simulink model "stateObserverControl"  (R2023b)
settings: Solver=VariableStepAuto  StartTime=0.0  StopTime=10  RelTol=1e-3
values from neighbouring files (symbols this model uses):
  K = Kaug(1:length(A))    [Controller.m]
  Km = Kaug(length(A)+1:end)    [Controller.m]
  L = place(A',C',poles)'    [Controller.m]
  Ma = [0 , 1 ; -1, 2*cos(w0)]    [Controller.m]
  Mb = [0;1]    [Controller.m]
  sys_est_ss = ss(A,B,C,D,Ts)    [Controller.m]
  Ts = 1/fs    (= 5e-05)    [Controller.m]
libraries: simulink x1
settings Model: Creator=NCS  LastModifiedBy=NCS

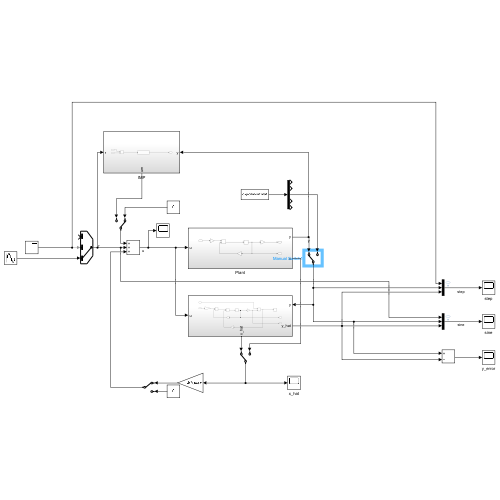
[thumbnail: Simulink's stored preview of the top-level diagram]
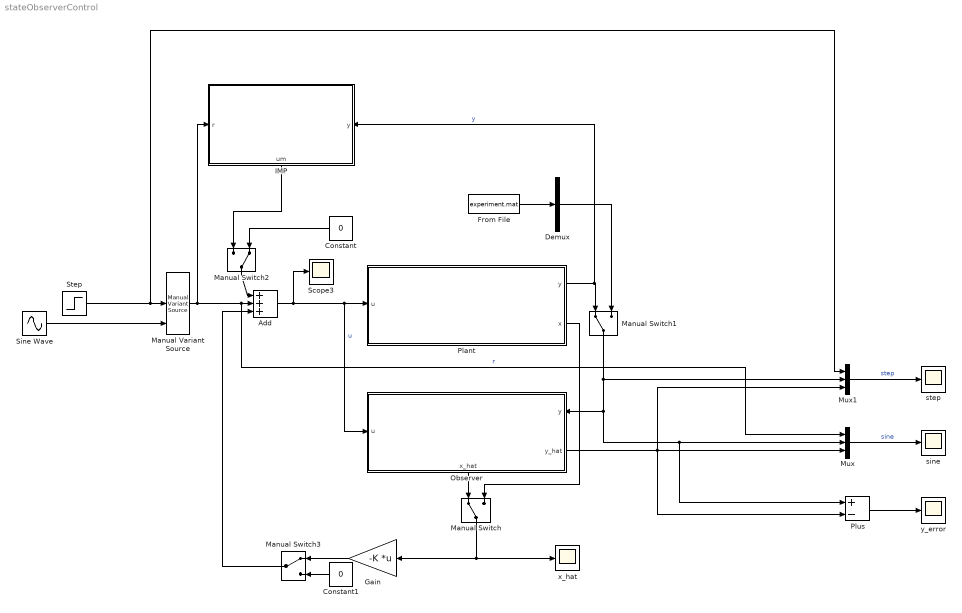
== system stateObserverControl ==
  Add : Sum  Inputs=+++
  Constant : Constant  Value=0
  Constant1 : Constant  Value=0
  Demux : Demux  Outputs=5
  From File : FromFile  FileName=experiment.mat  SampleTime=0
  Gain : Gain  Gain=-K  Multiplication=Matrix(K*u) (u vector)
  IMP : Subsystem
      settings: PortSchema="{\"entries\":[{\"content\":{\"sides\":[{\"content\":{\"connectorIds\":[\"In1\"]},\"type\":\"ConnectorPlacement.EquallySpacedRectSide\",\"uuid\":\"5d5e4b93-0997-4cc6-bb38-a0bc2c16a1b8\"},{\"content\":{\"connectorIds\":[\"In2\"],\"side\":\"RIGHT\"},\"type\":\"ConnectorPlacement.EquallySpacedRectSide\",\"uuid\":\"6a4a0bd4-0b0e-4fe8-aac6-62d10dbc348f\"},{\"content\":{\"side\":\"TOP\"},\"type\":\"ConnectorPlacement.EquallySpacedRectSide\",\"uuid\":\"dff729df-3d3e-4d9e-a17d-f1c4cc3cc1b7\"},{\"content\":{\"connectorIds\":[\"Out1\"],\"side\":\"BOTTOM\"},\"type\":\"ConnectorPlacement.EquallySpacedRectSide\",\"uuid\":\"a2ceeb7c-1f2e-4c64-a024-e96d715f5345\"}]},\"type\":\"ConnectorPlacement.EquallySpacedConnector\",\"uuid\":\"173e3c82-e772-4c04-9f4e-952750faad31\"}],\"packageUris\":[\"http://schema.mathworks.com/mf0/Connector/R2020b\"],\"version\":\"1.0\"}"
  Manual Variant Source : simulink/Signal Routing/Manual Variant Source  NumChoices=3  LabelModeActiveChoice=V_3
  Manual Switch : ManualSwitch
  Manual Switch1 : ManualSwitch
  Manual Switch2 : ManualSwitch  CurrentSetting=0
  Manual Switch3 : ManualSwitch
  Mux : Mux  Inputs=3
  Mux1 : Mux  Inputs=3
  Observer : Subsystem
      settings: PortSchema="{\"entries\":[{\"content\":{\"sides\":[{\"content\":{\"connectorIds\":[\"In1\",\"Out2\"]},\"type\":\"ConnectorPlacement.EquallySpacedRectSide\",\"uuid\":\"21983625-a237-4110-9725-a9924de32044\"},{\"content\":{\"connectorIds\":[\"In2\"],\"side\":\"RIGHT\"},\"type\":\"ConnectorPlacement.EquallySpacedRectSide\",\"uuid\":\"23fbd554-84a6-40c4-ba63-b021a939aeab\"},{\"content\":{\"side\":\"TOP\"},\"type\":\"ConnectorPlacement.EquallySpacedRectSide\",\"uuid\":\"d2b950d8-6865-452b-b7d3-0dc4efb78d1c\"},{\"content\":{\"connectorIds\":[\"Out1\"],\"side\":\"BOTTOM\"},\"type\":\"ConnectorPlacement.EquallySpacedRectSide\",\"uuid\":\"ad593450-6de1-4a85-9c80-0441fd99563e\"}]},\"type\":\"ConnectorPlacement.EquallySpacedConnector\",\"uuid\":\"76fef15a-6568-482c-8925-66f28f29b553\"}],\"packageUris\":[\"http://schema.mathworks.com/mf0/Connector/R2020b\"],\"version\":\"1.0\"}"
  Plant : Subsystem
      settings: PortSchema="{\"entries\":[{\"content\":{\"sides\":[{\"content\":{\"connectorIds\":[\"Out1\",\"Out2\"]},\"type\":\"ConnectorPlacement.EquallySpacedRectSide\",\"uuid\":\"21983625-a237-4110-9725-a9924de32044\"},{\"content\":{\"connectorIds\":[\"In1\"],\"side\":\"RIGHT\"},\"type\":\"ConnectorPlacement.EquallySpacedRectSide\",\"uuid\":\"23fbd554-84a6-40c4-ba63-b021a939aeab\"},{\"content\":{\"side\":\"TOP\"},\"type\":\"ConnectorPlacement.EquallySpacedRectSide\",\"uuid\":\"d2b950d8-6865-452b-b7d3-0dc4efb78d1c\"},{\"content\":{\"side\":\"BOTTOM\"},\"type\":\"ConnectorPlacement.EquallySpacedRectSide\",\"uuid\":\"ad593450-6de1-4a85-9c80-0441fd99563e\"}]},\"type\":\"ConnectorPlacement.EquallySpacedConnector\",\"uuid\":\"76fef15a-6568-482c-8925-66f28f29b553\"}],\"packageUris\":[\"http://schema.mathworks.com/mf0/Connector/R2020b\"],\"version\":\"1.0\"}"
  Plus : Sum  Inputs=+-
  Scope3 : Scope
  Sine Wave : Sin  Amplitude=0.2  Frequency=400*2*pi  SampleTime=Ts
  Step : Step  Time=0  After=0.2  SampleTime=Ts
  sine : Scope
  step : Scope
  x_hat : Scope
  y_error : Scope
  wires:
  Plant/1(y) -> Manual Switch1/1, IMP/2(y)  "y"
  Add/1 -> Plant/1(u), Observer/2(u), Scope3/1  "u"
  Observer/1(x_hat) -> Manual Switch/1
  Plant/2(x) -> Manual Switch/2
  Manual Switch/1 -> x_hat/1, Gain/1
  Sine Wave/1 -> Manual Variant Source/3
  Manual Variant Source/1 -> IMP/1(r), Mux/1, Add/2  "r"
  Step/1 -> Manual Variant Source/2, Mux1/1
  Mux/1 -> sine/1  "sine"
  Mux1/1 -> step/1  "step"
  Manual Switch2/1 -> Add/1
  IMP/1(um) -> Manual Switch2/1
  Constant/1 -> Manual Switch2/2
  Observer/2(y_hat) -> Mux1/3, Mux/3, Plus/2
  From File/1 -> Demux/1
  Demux/3 -> Manual Switch1/2
  Manual Switch1/1 -> Mux1/2, Mux/2, Plus/1, Observer/1(y)
  Manual Switch3/1 -> Add/3
  Gain/1 -> Manual Switch3/1
  Constant1/1 -> Manual Switch3/2
  Plus/1 -> y_error/1

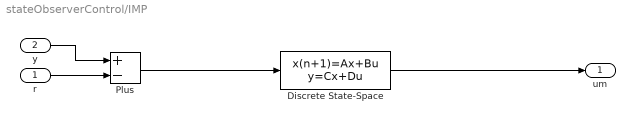
== system stateObserverControl/IMP ==
  r : Inport
  y : Inport  Port=2
  Discrete State-Space : DiscreteStateSpace  A=Ma  B=Mb  C=-Km  D=0  SampleTime=-1
  Plus : Sum  Inputs=+-
  um : Outport
  wires:
  Plus/1 -> Discrete State-Space/1
  Discrete State-Space/1 -> um/1
  y/1 -> Plus/1
  r/1 -> Plus/2

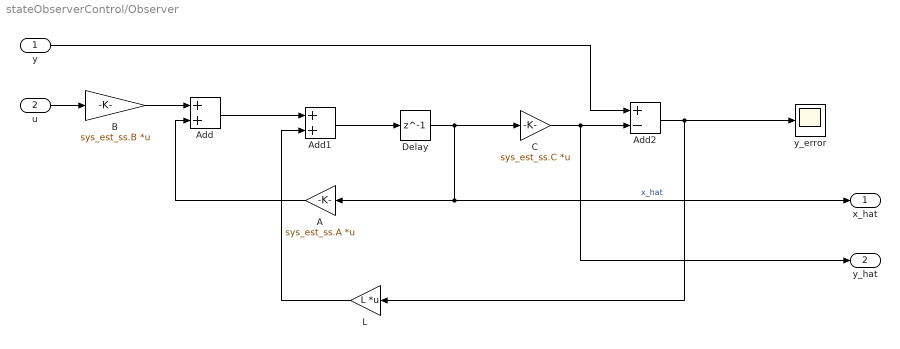
== system stateObserverControl/Observer ==
  y : Inport
  u : Inport  Port=2
  A : Gain  Gain=sys_est_ss.A  Multiplication=Matrix(K*u) (u vector)
  Add : Sum
  Add1 : Sum
  Add2 : Sum  Inputs=+-
  B : Gain  Gain=sys_est_ss.B  Multiplication=Matrix(K*u) (u vector)
  C : Gain  Gain=sys_est_ss.C  Multiplication=Matrix(K*u) (u vector)
  Delay : Delay  DelayLength=1  InitialCondition=1
  L : Gain  Gain=L  Multiplication=Matrix(K*u) (u vector)
  y_error : Scope
  x_hat : Outport
  y_hat : Outport  Port=2
  wires:
  B/1 -> Add/1
  u/1 -> B/1
  Add/1 -> Add1/1
  Add1/1 -> Delay/1
  Delay/1 -> C/1, x_hat/1, A/1  "x_hat"
  A/1 -> Add/2
  y/1 -> Add2/1
  C/1 -> y_hat/1, Add2/2
  Add2/1 -> y_error/1, L/1
  L/1 -> Add1/2

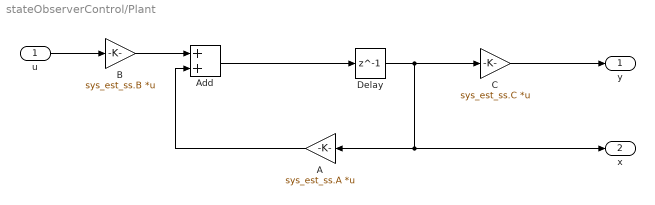
== system stateObserverControl/Plant ==
  u : Inport
  A : Gain  Gain=sys_est_ss.A  Multiplication=Matrix(K*u) (u vector)
  Add : Sum
  B : Gain  Gain=sys_est_ss.B  Multiplication=Matrix(K*u) (u vector)
  C : Gain  Gain=sys_est_ss.C  Multiplication=Matrix(K*u) (u vector)
  Delay : Delay  DelayLength=1  InitialCondition=0
  y : Outport
  x : Outport  Port=2
  wires:
  B/1 -> Add/1
  u/1 -> B/1
  Add/1 -> Delay/1
  Delay/1 -> x/1, A/1, C/1
  A/1 -> Add/2
  C/1 -> y/1
